simulink model "second_cl_2_clean"  (R2021a)
settings: Solver=VariableStepAuto  StartTime=0.0  StopTime=20  RelTol=1e-3
values from neighbouring files (symbols this model uses):
  dist = [0;dist_theta;0;0]    [ex3main.m]
  K = lqr(sys,Q,R)    [ex3main.m]
  params = get_params()    [ex3main.m]
  sys = get_system(params)    [ex3main.m]
  Ts = 1/200    (= 0.005)    [ex3main.m]
  wc = 2*f*pi    (= 18.8495559215)    [ex3main.m]
libraries: simulink x2
settings Model: Creator=martijndebeuf  LastModifiedBy=martijndebeuf
settings SolverCC: AlgebraicLoopSolver=TrustRegion
settings DebuggingCC: SFMachineParentedDataDiag=warning

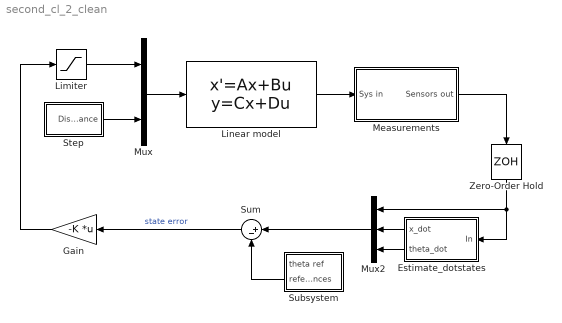
== system second_cl_2_clean ==
  Estimate_dotstates : Subsystem
  Gain : Gain  Gain=-K  Multiplication=Matrix(K*u) (u vector)
  Limiter : Saturate  UpperLimit=5  LowerLimit=-5
  Linear model : StateSpace  A=sys.A  B=[sys.B,dist]  C=sys.C  D=[sys.D,zeros(2,1)]  InitialCondition=initial_conditions'
  Measurements : Subsystem
  Mux : Mux  Inputs=2
  Mux2 : Mux  Inputs=3
  Step : Subsystem
  Subsystem : Subsystem
  Sum : Sum  Inputs=|+-
  Zero-Order Hold : ZeroOrderHold  SampleTime=Ts
  wires:
  Mux/1 -> Linear model/1
  Limiter/1 -> Mux/1
  Gain/1 -> Limiter/1
  Sum/1 -> Gain/1  "state error"
  Mux2/1 -> Sum/1
  Step/1(Disturbance) -> Mux/2
  Estimate_dotstates/1(x_dot) -> Mux2/2
  Estimate_dotstates/2(theta_dot) -> Mux2/3
  Linear model/1 -> Measurements/1(" Sys in")
  Measurements/1(Sensors out) -> Zero-Order Hold/1
  Subsystem/2(references) -> Sum/2
  Zero-Order Hold/1 -> Mux2/1, Estimate_dotstates/1(In)

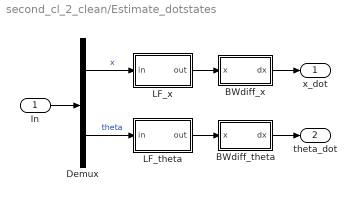
== system second_cl_2_clean/Estimate_dotstates ==
  In : Inport
  BWdiff_theta : Subsystem
  BWdiff_x : Subsystem
  Demux : Demux  Outputs=2
  LF_theta : Subsystem
  LF_x : Subsystem
  x_dot : Outport
  theta_dot : Outport  Port=2
  wires:
  LF_theta/1(out) -> BWdiff_theta/1(x)
  Demux/2 -> LF_theta/1(in)  "theta"
  BWdiff_theta/1(dx) -> theta_dot/1
  BWdiff_x/1(dx) -> x_dot/1
  Demux/1 -> LF_x/1(in)  "x"
  In/1 -> Demux/1
  LF_x/1(out) -> BWdiff_x/1(x)

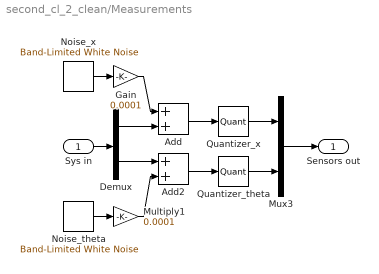
== system second_cl_2_clean/Measurements ==
  " Sys in" : Inport
  Add : Sum
  Add2 : Sum
  Demux : Demux  Outputs=2
  Gain : Gain  Gain=0.0001
  Multiply1 : Gain  Gain=0.0001
  Mux3 : Mux  Inputs=2
  Noise_theta : simulink/Sources/Band-Limited White Noise  Cov=[0.1]  Ts=Ts  seed=[23342]
  Noise_x : simulink/Sources/Band-Limited White Noise  Cov=[0.1]  Ts=Ts  seed=[23341]
  Quantizer_theta : Quantizer  QuantizationInterval=resolutiontheta
  Quantizer_x : Quantizer  QuantizationInterval=resolutionx
  Sensors out : Outport
  wires:
  " Sys in"/1 -> Demux/1
  Gain/1 -> Add/1
  Multiply1/1 -> Add2/2
  Add2/1 -> Quantizer_theta/1
  Noise_theta/1 -> Multiply1/1
  Mux3/1 -> Sensors out/1
  Quantizer_x/1 -> Mux3/1
  Demux/2 -> Add2/1
  Demux/1 -> Add/2
  Add/1 -> Quantizer_x/1
  Quantizer_theta/1 -> Mux3/2
  Noise_x/1 -> Gain/1

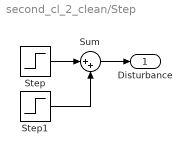
== system second_cl_2_clean/Step ==
  Step : Step  Time=3  SampleTime=Ts
  Step1 : Step  Time=3.1  SampleTime=Ts
  Sum : Sum  Inputs=|++
  Disturbance : Outport
  wires:
  Step/1 -> Sum/1
  Step1/1 -> Sum/2
  Sum/1 -> Disturbance/1

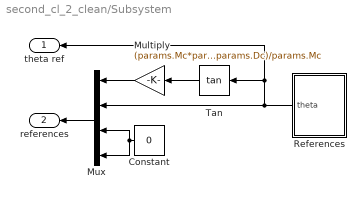
== system second_cl_2_clean/Subsystem ==
  Constant : Constant  Value=0
  Multiply : Gain  Gain=(params.Mc*params.Dt+params.Msw*params.Dc)/params.Mc
  Mux : Mux
  References : Subsystem
  Tan : Trigonometry  Operator=tan
  theta ref : Outport
  references : Outport  Port=2
  wires:
  Mux/1 -> references/1
  Tan/1 -> Multiply/1
  Multiply/1 -> Mux/1
  References/1(theta) -> Mux/2, Tan/1, theta ref/1
  Constant/1 -> Mux/4, Mux/3

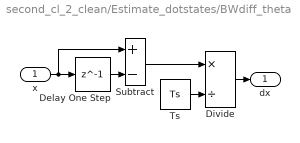
== system second_cl_2_clean/Estimate_dotstates/BWdiff_theta ==
  x : Inport
  Delay One Step : Delay  DelayLength=1
  Divide : Product  Inputs=*/
  Subtract : Sum  Inputs=+-
  Ts : Constant  Value=Ts
  dx : Outport
  wires:
  Ts/1 -> Divide/2
  Subtract/1 -> Divide/1
  x/1 -> Delay One Step/1, Subtract/1
  Divide/1 -> dx/1
  Delay One Step/1 -> Subtract/2

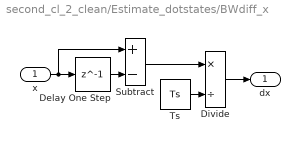
== system second_cl_2_clean/Estimate_dotstates/BWdiff_x ==
  x : Inport
  Delay One Step : Delay  DelayLength=1
  Divide : Product  Inputs=*/
  Subtract : Sum  Inputs=+-
  Ts : Constant  Value=Ts
  dx : Outport
  wires:
  Ts/1 -> Divide/2
  Subtract/1 -> Divide/1
  x/1 -> Delay One Step/1, Subtract/1
  Divide/1 -> dx/1
  Delay One Step/1 -> Subtract/2

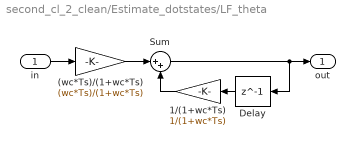
== system second_cl_2_clean/Estimate_dotstates/LF_theta ==
  in : Inport
  (wc*Ts)/(1+wc*Ts) : Gain  Gain=(wc*Ts)/(1+wc*Ts)
  1/(1+wc*Ts) : Gain  Gain=1/(1+wc*Ts)
  Delay : Delay  DelayLength=1
  Sum : Sum  Inputs=|++
  out : Outport
  wires:
  1/(1+wc*Ts)/1 -> Sum/2
  Sum/1 -> out/1, Delay/1
  (wc*Ts)/(1+wc*Ts)/1 -> Sum/1
  in/1 -> (wc*Ts)/(1+wc*Ts)/1
  Delay/1 -> 1/(1+wc*Ts)/1

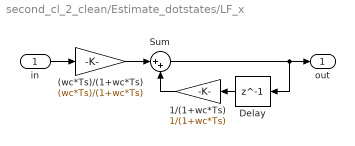
== system second_cl_2_clean/Estimate_dotstates/LF_x ==
  in : Inport
  (wc*Ts)/(1+wc*Ts) : Gain  Gain=(wc*Ts)/(1+wc*Ts)
  1/(1+wc*Ts) : Gain  Gain=1/(1+wc*Ts)
  Delay : Delay  DelayLength=1
  Sum : Sum  Inputs=|++
  out : Outport
  wires:
  1/(1+wc*Ts)/1 -> Sum/2
  Sum/1 -> out/1, Delay/1
  (wc*Ts)/(1+wc*Ts)/1 -> Sum/1
  in/1 -> (wc*Ts)/(1+wc*Ts)/1
  Delay/1 -> 1/(1+wc*Ts)/1

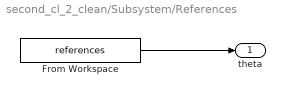
== system second_cl_2_clean/Subsystem/References ==
  From Workspace : FromWorkspace  VariableName=references  SampleTime=Ts  Interpolate=off  OutputAfterFinalValue=Holding final value
  theta : Outport
  wires:
  From Workspace/1 -> theta/1
